simulink model "Template_v3_08_2020a"  (R2020a)
settings: Solver=FixedStepAuto  StartTime=0.0  StopTime=tsim  FixedStep=baseRate  MaxStep=0.0001  RelTol=1e-6  AbsTol=1e-6  EnableMultiTasking=on
values from neighbouring files (symbols this model uses):
  baseRate = 0.05    [Run_Initializer.m]
  drop_states_ARM = [ pi/2, pi/2, 0]    [Run_Initializer.m]
  drop_states_BLACK = [ xLength/2, yLength/2, 0]    [Run_Initializer.m]
  drop_states_BLUE = [ xLength/2-0.5; yLength/2; 0]    [Run_Initializer.m]
  drop_states_RED = [ xLength/2+0.5, yLength/2, pi]    [Run_Initializer.m]
  F_Black_X_nominal = 0.2196    [Run_Initializer.m]
  F_Black_Y_nominal = 0.2825    [Run_Initializer.m]
  F_Blue_X_nominal = 0.2196    [Run_Initializer.m]
  F_Blue_Y_nominal = 0.2825    [Run_Initializer.m]
  F_red_X_nominal = 0.2196    [Run_Initializer.m]
  F_red_Y_nominal = 0.2825    [Run_Initializer.m]
  F_thrusters_BLACK = [F_Black_X_nominal; F_Black_X_nominal;                             F_Black_Y_nominal; F_Black_Y_nominal; F_Black_X_nominal;                              F_Black_X_nominal; F_Black_Y_nominal; F_Black_Y_nominal]    [Run_Initializer.m]
  F_thrusters_BLUE = [F_Blue_X_nominal; F_Blue_X_nominal;                             F_Blue_Y_nominal; F_Blue_Y_nominal; F_Blue_X_nominal;                              F_Blue_X_nominal; F_Blue_Y_nominal; F_Blue_Y_nominal]    [Run_Initializer.m]
  F_thrusters_RED = [F_red_X_nominal; F_red_X_nominal;                             F_red_Y_nominal; F_red_Y_nominal; F_red_X_nominal;                              F_red_X_nominal; F_red_Y_nominal; F_red_Y_nominal]    [Run_Initializer.m]
  Gamma1_el = 0.12    [Run_Initializer.m]
  Gamma1_sh = 0.005    [Run_Initializer.m]
  Gamma1_wr = 0.025    [Run_Initializer.m]
  Gamma2_el = 5    [Run_Initializer.m]
  Gamma2_sh = 15    [Run_Initializer.m]
  Gamma2_wr = 5    [Run_Initializer.m]
  Gamma3_el = 10    [Run_Initializer.m]
  Gamma3_sh = 40    [Run_Initializer.m]
  Gamma3_wr = 40    [Run_Initializer.m]
  Gamma4_el = 0.039    [Run_Initializer.m]
  Gamma4_sh = 0.015    [Run_Initializer.m]
  Gamma4_wr = 0.029    [Run_Initializer.m]
  Gamma5_el = 800    [Run_Initializer.m]
  Gamma5_sh = 800    [Run_Initializer.m]
  Gamma5_wr = 800    [Run_Initializer.m]
  Gamma6_el = 0.000001    (= 1e-06)    [Run_Initializer.m]
  Gamma6_sh = 0.005    [Run_Initializer.m]
  Gamma6_wr = 0.02    [Run_Initializer.m]
  home_states_BLACK = [ xLength/2; yLength/2; 0]    [Run_Initializer.m]
  home_states_BLUE = [ xLength/2-0.9; yLength/2; 0]    [Run_Initializer.m]
  home_states_RED = [ xLength/2+0.9; yLength/2; pi]    [Run_Initializer.m]
  init_states_BLACK = [ xLength/2; yLength/2; 0]    [Run_Initializer.m]
  init_states_BLUE = [ xLength/2-0.9; yLength/2; 0]    [Run_Initializer.m]
  init_states_RED = [ xLength/2+0.9; yLength/2; pi]    [Run_Initializer.m]
  Kd_tb = 1.0    (= 1)    [Run_Initializer.m]
  Kd_tblue = 1    [Run_Initializer.m]
  Kd_tr = 1.0    (= 1)    [Run_Initializer.m]
  Kd_xb = 8    [Run_Initializer.m]
  Kd_xblue = 8    [Run_Initializer.m]
  Kd_xr = 8    [Run_Initializer.m]
  Kd_yb = 8    [Run_Initializer.m]
  Kd_yblue = 8    [Run_Initializer.m]
  Kd_yr = 8    [Run_Initializer.m]
  Kp_tb = 0.1    [Run_Initializer.m]
  Kp_tblue = 0.1    [Run_Initializer.m]
  Kp_tr = 0.1    [Run_Initializer.m]
  Kp_xb = 2    [Run_Initializer.m]
  Kp_xblue = 2    [Run_Initializer.m]
  Kp_xr = 2    [Run_Initializer.m]
  Kp_yb = 2    [Run_Initializer.m]
  Kp_yblue = 2    [Run_Initializer.m]
  Kp_yr = 2    [Run_Initializer.m]
  noise_variance_BLACK = 0    [Run_Initializer.m]
  noise_variance_BLUE = 0    [Run_Initializer.m]
  noise_variance_RED = 0    [Run_Initializer.m]
  Phase0_End = Phase0_Duration    (= 10)    [Run_Initializer.m]
  Phase1_End = Phase0_Duration + Phase1_Duration    (= 15)    [Run_Initializer.m]
  Phase2_End = Phase0_Duration + Phase1_Duration +                                   Phase2_Duration    (= 35)    [Run_Initializer.m]
  Phase3_End = Phase0_Duration + Phase1_Duration +                                   Phase2_Duration + Phase3_Duration    (= 155)    [Run_Initializer.m]
  Phase3_SubPhase1_End = Phase2_End + Phase3_SubPhase1_Duration    (= 155)    [Run_Initializer.m]
  Phase3_SubPhase2_End = Phase2_End + Phase3_SubPhase1_Duration +                                   Phase3_SubPhase2_Duration    (= 155)    [Run_Initializer.m]
  Phase3_SubPhase3_End = Phase2_End + Phase3_SubPhase1_Duration +                                   Phase3_SubPhase2_Duration +                                  Phase3_SubPhase3_Duration    (= 155)    [Run_Initializer.m]
  Phase3_SubPhase4_End = Phase2_End + Phase3_SubPhase1_Duration +                                   Phase3_SubPhase2_Duration +                                  Phase3_SubPhase3_Duration +                                  Phase3_SubPhase4_Duration    [Run_Initializer.m]
  Phase4_End = Phase0_Duration + Phase1_Duration +                                   Phase2_Duration + Phase3_Duration +                                   Phase4_Duration    (= 275)    [Run_Initializer.m]
  Phase5_End = Phase0_Duration + Phase1_Duration +                                   Phase2_Duration + Phase3_Duration +                                   Phase4_Duration + Phase5_Duration    (= 295)    [Run_Initializer.m]
  thruster_dist2CG_BLACK = [72.80;-65.20;61.75;-79.75;65.20;-65.20;74.25;-54.75]    [Run_Initializer.m]
  thruster_dist2CG_BLUE = [83.10;-54.90;71.50;-70.00;54.90;-75.50;64.50;-64.50]    [Run_Initializer.m]
  thruster_dist2CG_RED = [69.38;-56.62;50.01;-81.49;61.12;-68.38;78.99;-52.01]    [Run_Initializer.m]
  Tz_lim_elarm = .1    (= 0.1)    [Run_Initializer.m]
  Tz_lim_sharm = .1    (= 0.1)    [Run_Initializer.m]
  Tz_lim_wrarm = .1    (= 0.1)    [Run_Initializer.m]
  xLength = 3.51155    [Run_Initializer.m]
  yLength = 2.41935    [Run_Initializer.m]
undefined symbols (not defined in the file or in its folder): b0, b1, b_out, CHASER_ABSOLUTE_POSITION, DiscIntNeverNeededParam, MAX_BODY_ANGULAR_VELOCITY, MAX_VELOCITY, model_param, platformSelection, relevant_half_range, relevant_state_mean, serverRate, simMode, w0, w1, w_out
libraries: dspstat3 x18, raspberrypiBasiclib x9, dspsigops x9, embdlinuxlib x7, simulink x7, MainLibrary x4, mspfiltlib x3, dsparch4 x3, etargetslib x1, sensehatlib x1
(part 3 of 12)

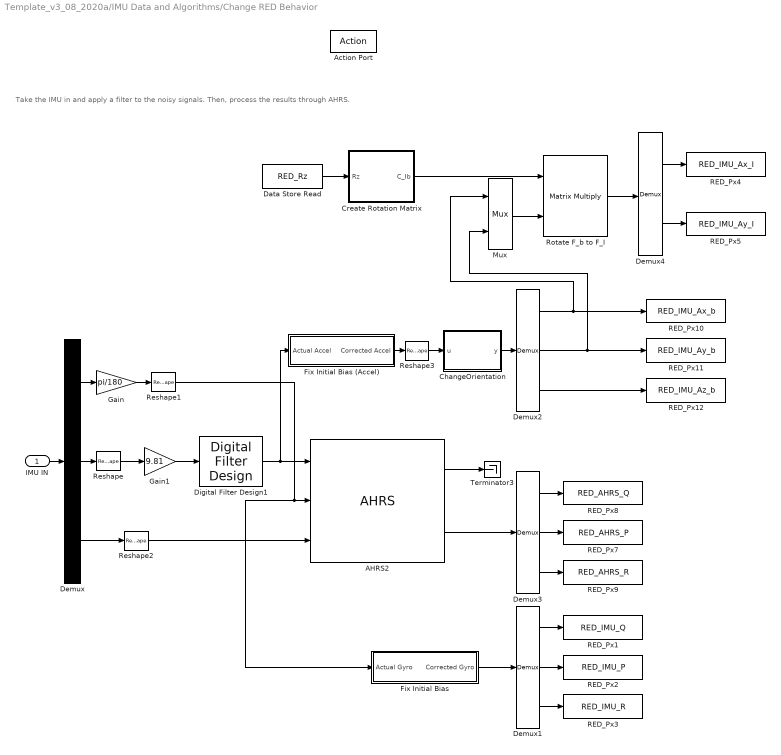
== system Template_v3_08_2020a/IMU Data and Algorithms/Change RED Behavior ==
  note: Take the IMU in and apply a filter to the noisy signals. Then, process the results through AHRS.
  IMU IN : Inport
  Action Port : ActionPort  ActionPortLabel=if(u1 == 1 & u2 ==0)
  AHRS2 : mspfiltlib/AHRS  DispRefFrame=NED  DecimationFactor=1  InitialProcessNoise=ahrsfilter.defaultProcessNoise  OrientationFormat=quaternion  SimulateUsing=Interpreted execution  AccelerometerNoise=0.0001924722  GyroscopeNoise=9.1385e-5  MagnetometerNoise=0.1  GyroscopeDriftNoise=3.0462e-13  LinearAccelerationNoise=0.0096236100000000012  MagneticDisturbanceNoise=0.5  LinearAccelerationDecayFactor=0.5  MagneticDisturbanceDecayFactor=0.5  ExpectedMagneticFieldStrength=33
      settings: SourceProductBaseCode=TF,NV
  ChangeOrientation : MATLAB Function  TreatAsAtomicUnit=on
  Create Rotation Matrix : MATLAB Function  TreatAsAtomicUnit=on
  Data Store Read : DataStoreRead  DataStoreName=RED_Rz
  Demux : Demux  Outputs=[3,3,3]
  Demux1 : Demux  Outputs=3
  Demux2 : Demux  Outputs=3
  Demux3 : Demux  Outputs=3
  Demux4 : Demux  Outputs=2
  Digital Filter Design1 : dsparch4/Digital Filter Design  mwdsp_browser_bugfix_var=off
  Fix Initial Bias : Subsystem
  Fix Initial Bias (Accel) : Subsystem
  Gain : Gain  Gain=pi/180
  Gain1 : Gain  Gain=9.81
  Mux : Mux  Inputs=2
  RED_Px1 : DataStoreWrite  DataStoreName=RED_IMU_Q
  RED_Px10 : DataStoreWrite  DataStoreName=RED_IMU_Ax_b
  RED_Px11 : DataStoreWrite  DataStoreName=RED_IMU_Ay_b
  RED_Px12 : DataStoreWrite  DataStoreName=RED_IMU_Az_b
  RED_Px2 : DataStoreWrite  DataStoreName=RED_IMU_P
  RED_Px3 : DataStoreWrite  DataStoreName=RED_IMU_R
  RED_Px4 : DataStoreWrite  DataStoreName=RED_IMU_Ax_I
  RED_Px5 : DataStoreWrite  DataStoreName=RED_IMU_Ay_I
  RED_Px7 : DataStoreWrite  DataStoreName=RED_AHRS_P
  RED_Px8 : DataStoreWrite  DataStoreName=RED_AHRS_Q
  RED_Px9 : DataStoreWrite  DataStoreName=RED_AHRS_R
  Reshape{,1..3} (4 alike) : Reshape  OutputDimensionality=Row vector (2-D)
  Rotate F_b to F_I : Product  Multiplication=Matrix(*)
  Terminator3 : Terminator
  wires:
  Reshape2/1 -> AHRS2/3
  Gain/1 -> Reshape1/1
  Demux2/3 -> RED_Px12/1
  Demux3/3 -> RED_Px9/1
  AHRS2/2 -> Demux3/1
  AHRS2/1 -> Terminator3/1
  Reshape/1 -> Gain1/1
  Demux/2 -> Reshape/1
  Demux/3 -> Reshape2/1
  Demux/1 -> Gain/1
  IMU IN/1 -> Demux/1
  Demux1/1 -> RED_Px1/1
  Demux1/2 -> RED_Px2/1
  Demux1/3 -> RED_Px3/1
  Fix Initial Bias/1(Corrected Gyro) -> Demux1/1
  ChangeOrientation/1(y) -> Demux2/1
  Demux3/2 -> RED_Px7/1
  Demux3/1 -> RED_Px8/1
  Digital Filter Design1/1 -> Fix Initial Bias (Accel)/1(Actual Accel), AHRS2/1
  Gain1/1 -> Digital Filter Design1/1
  Reshape3/1 -> ChangeOrientation/1(u)
  Fix Initial Bias (Accel)/1(Corrected Accel) -> Reshape3/1
  Reshape1/1 -> Fix Initial Bias/1(Actual Gyro), AHRS2/2
  Data Store Read/1 -> Create Rotation Matrix/1(Rz)
  Mux/1 -> Rotate F_b to F_I/2
  Rotate F_b to F_I/1 -> Demux4/1
  Create Rotation Matrix/1(C_Ib) -> Rotate F_b to F_I/1
  Demux2/2 -> Mux/2, RED_Px11/1
  Demux4/1 -> RED_Px4/1
  Demux4/2 -> RED_Px5/1
  Demux2/1 -> Mux/1, RED_Px10/1

== system Template_v3_08_2020a/IMU Data and Algorithms/Is this a simulation? ==
  Constant : Constant  Value=simMode  SampleTime=-1
  isSim : Outport  VectorParamsAs1DForOutWhenUnconnected=off
  wires:
  Constant/1 -> isSim/1

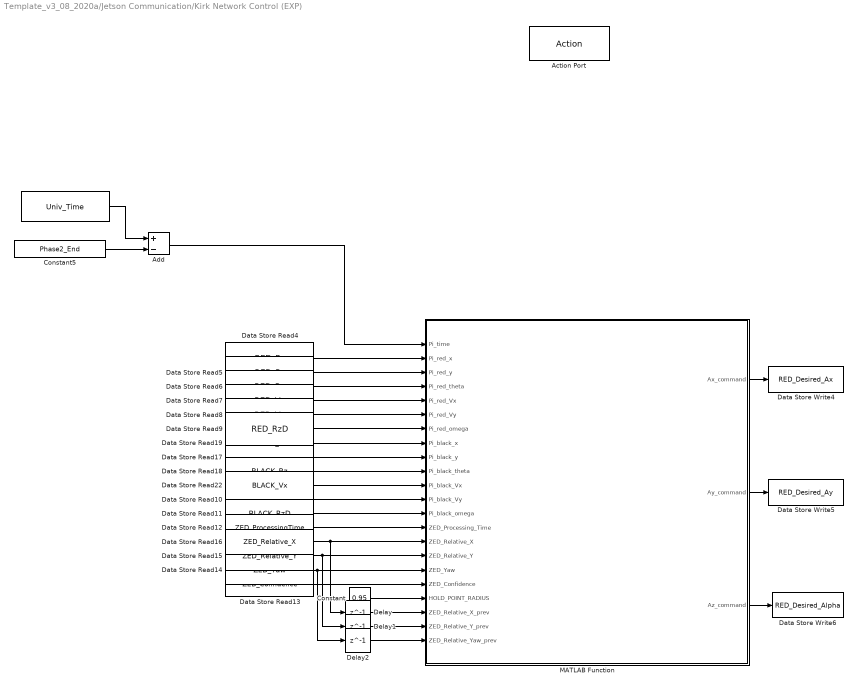
== system Template_v3_08_2020a/Jetson Communication/Kirk Network Control (EXP) ==
  Action Port : ActionPort  ActionPortLabel=if((u1 == 1 & u2 == 0) & (u3 > u4) & (u3 < u5) )
  " " : DataStoreRead  DataStoreName=Univ_Time
  Add : Sum  Inputs=+-
  Constant : Constant  Value=0.95
  Constant5 : Constant  Value=Phase2_End
  Data Store Read10 : DataStoreRead  DataStoreName=BLACK_Vy
  Data Store Read11 : DataStoreRead  DataStoreName=BLACK_RzD
  Data Store Read12 : DataStoreRead  DataStoreName=ZED_ProcessingTime
  Data Store Read13 : DataStoreRead  DataStoreName=ZED_Confidence
  Data Store Read14 : DataStoreRead  DataStoreName=ZED_Yaw
  Data Store Read15 : DataStoreRead  DataStoreName=ZED_Relative_Y
  Data Store Read16 : DataStoreRead  DataStoreName=ZED_Relative_X
  Data Store Read17 : DataStoreRead  DataStoreName=BLACK_Py
  Data Store Read18 : DataStoreRead  DataStoreName=BLACK_Rz
  Data Store Read19 : DataStoreRead  DataStoreName=BLACK_Px
  Data Store Read22 : DataStoreRead  DataStoreName=BLACK_Vx
  Data Store Read4 : DataStoreRead  DataStoreName=RED_Px
  Data Store Read5 : DataStoreRead  DataStoreName=RED_Py
  Data Store Read6 : DataStoreRead  DataStoreName=RED_Rz
  Data Store Read7 : DataStoreRead  DataStoreName=RED_Vx
  Data Store Read8 : DataStoreRead  DataStoreName=RED_Vy
  Data Store Read9 : DataStoreRead  DataStoreName=RED_RzD
  Data Store Write4 : DataStoreWrite  DataStoreName=RED_Desired_Ax
  Data Store Write5 : DataStoreWrite  DataStoreName=RED_Desired_Ay
  Data Store Write6 : DataStoreWrite  DataStoreName=RED_Desired_Alpha
  Delay : Delay  DelayLength=1
  Delay1 : Delay  DelayLength=1
  Delay2 : Delay  DelayLength=1
  MATLAB Function : MATLAB Function  TreatAsAtomicUnit=on
  wires:
  Data Store Read11/1 -> MATLAB Function/13(Pi_black_omega)
  Data Store Read7/1 -> MATLAB Function/5(Pi_red_Vx)
  " "/1 -> Add/1
  Data Store Read18/1 -> MATLAB Function/10(Pi_black_theta)
  Data Store Read17/1 -> MATLAB Function/9(Pi_black_y)
  Data Store Read8/1 -> MATLAB Function/6(Pi_red_Vy)
  MATLAB Function/2(Ay_command) -> Data Store Write5/1
  Data Store Read10/1 -> MATLAB Function/12(Pi_black_Vy)
  Data Store Read22/1 -> MATLAB Function/11(Pi_black_Vx)
  Data Store Read19/1 -> MATLAB Function/8(Pi_black_x)
  Data Store Read5/1 -> MATLAB Function/3(Pi_red_y)
  Add/1 -> MATLAB Function/1(Pi_time)
  Data Store Read9/1 -> MATLAB Function/7(Pi_red_omega)
  Constant5/1 -> Add/2
  Data Store Read15/1 -> MATLAB Function/16(ZED_Relative_Y), Delay1/1
  Data Store Read13/1 -> MATLAB Function/18(ZED_Confidence)
  MATLAB Function/3(Az_command) -> Data Store Write6/1
  Data Store Read12/1 -> MATLAB Function/14(ZED_Processing_Time)
  MATLAB Function/1(Ax_command) -> Data Store Write4/1
  Data Store Read6/1 -> MATLAB Function/4(Pi_red_theta)
  Data Store Read4/1 -> MATLAB Function/2(Pi_red_x)
  Data Store Read16/1 -> Delay/1, MATLAB Function/15(ZED_Relative_X)
  Data Store Read14/1 -> Delay2/1, MATLAB Function/17(ZED_Yaw)
  Constant/1 -> MATLAB Function/19(HOLD_POINT_RADIUS)
  Delay/1 -> MATLAB Function/20(ZED_Relative_X_prev)
  Delay1/1 -> MATLAB Function/21(ZED_Relative_Y_prev)
  Delay2/1 -> MATLAB Function/22(ZED_Relative_Yaw_prev)

== system Template_v3_08_2020a/Jetson Communication/Kirk Network Control (SIM) ==
  Action Port : ActionPort  ActionPortLabel=elseif((u2 == 1) & (u3 > u4) & (u3 < u5) )
  " " : DataStoreRead  DataStoreName=Univ_Time
  Add : Sum  Inputs=+-
  Constant : Constant  Value=0.95
  Constant5 : Constant  Value=Phase2_End
  Data Store Read : DataStoreRead  DataStoreName=RED_Px
  Data Store Read1 : DataStoreRead  DataStoreName=RED_Py
  Data Store Read10 : DataStoreRead  DataStoreName=BLACK_Vy
  Data Store Read11 : DataStoreRead  DataStoreName=BLACK_RzD
  Data Store Read17 : DataStoreRead  DataStoreName=BLACK_Py
  Data Store Read18 : DataStoreRead  DataStoreName=BLACK_Rz
  Data Store Read2 : DataStoreRead  DataStoreName=RED_Rz
  Data Store Read22 : DataStoreRead  DataStoreName=BLACK_Vx
  Data Store Read6 : DataStoreRead  DataStoreName=RED_Vx
  Data Store Read7 : DataStoreRead  DataStoreName=RED_Vy
  Data Store Read8 : DataStoreRead  DataStoreName=RED_RzD
  Data Store Read9 : DataStoreRead  DataStoreName=BLACK_Px
  Data Store Write3 : DataStoreWrite  DataStoreName=RED_Desired_Ax
  Data Store Write4 : DataStoreWrite  DataStoreName=RED_Desired_Ay
  Data Store Write5 : DataStoreWrite  DataStoreName=RED_Desired_Alpha
  Delay : Delay  DelayLength=10
  Delay1 : Delay  DelayLength=10
  Delay2 : Delay  DelayLength=10
  MATLAB Function : MATLAB Function  TreatAsAtomicUnit=on
  Zero-Order Hold : ZeroOrderHold  SampleTime=0.5
  Zero-Order Hold1 : ZeroOrderHold  SampleTime=0.5
  Zero-Order Hold2 : ZeroOrderHold  SampleTime=0.5
  wires:
  Data Store Read1/1 -> MATLAB Function/3(Pi_red_y)
  Data Store Read/1 -> MATLAB Function/2(Pi_red_x)
  Data Store Read2/1 -> MATLAB Function/4(Pi_red_theta)
  Data Store Read9/1 -> Zero-Order Hold/1
  Data Store Read17/1 -> Zero-Order Hold1/1
  Data Store Read18/1 -> Zero-Order Hold2/1
  MATLAB Function/1(Ax_command) -> Data Store Write3/1
  MATLAB Function/2(Ay_command) -> Data Store Write4/1
  MATLAB Function/3(Az_command) -> Data Store Write5/1
  Data Store Read6/1 -> MATLAB Function/5(Pi_red_Vx)
  Data Store Read7/1 -> MATLAB Function/6(Pi_red_Vy)
  Data Store Read8/1 -> MATLAB Function/7(Pi_red_omega)
  Data Store Read22/1 -> MATLAB Function/11(Pi_black_Vx)
  Data Store Read10/1 -> MATLAB Function/12(Pi_black_Vy)
  Data Store Read11/1 -> MATLAB Function/13(Pi_black_omega)
  " "/1 -> Add/1
  Add/1 -> MATLAB Function/1(Pi_time)
  Constant5/1 -> Add/2
  Zero-Order Hold/1 -> Delay/1
  Zero-Order Hold1/1 -> Delay1/1
  Zero-Order Hold2/1 -> Delay2/1
  Constant/1 -> MATLAB Function/14(HOLD_POINT_RADIUS)
  Delay/1 -> MATLAB Function/8(Pi_black_x)
  Delay1/1 -> MATLAB Function/9(Pi_black_y)
  Delay2/1 -> MATLAB Function/10(Pi_black_theta)

== system Template_v3_08_2020a/Jetson Communication/isSim ==
  Constant : Constant  Value=simMode  SampleTime=-1
  isSim : Outport  VectorParamsAs1DForOutWhenUnconnected=off
  wires:
  Constant/1 -> isSim/1

== system Template_v3_08_2020a/Manipulator Encoder Data/Change Behavior ==
  Action Port : ActionPort  ActionPortLabel=if(u1 == 0)
  Data Store Write : DataStoreWrite  DataStoreName=RED_Rz_Shoulder
  Data Store Write1 : DataStoreWrite  DataStoreName=RED_Rz_Elbow
  Data Store Write2 : DataStoreWrite  DataStoreName=RED_Rz_Wrist
  Data Store Write3 : DataStoreWrite  DataStoreName=RED_RzD_Shoulder
  Data Store Write4 : DataStoreWrite  DataStoreName=RED_RzD_Elbow
  Data Store Write5 : DataStoreWrite  DataStoreName=RED_RzD_Wrist
  Read Joint Positions using Dynamixel Encoders : MainLibrary/Dynamixel Functions/Read Joint Positions using  Dynamixel Encoders  SampleTime=baseRate
      settings: SourceProductName=SPOT Custom Library
  wires:
  Read Joint Positions using Dynamixel Encoders/1 -> Data Store Write/1
  Read Joint Positions using Dynamixel Encoders/2 -> Data Store Write1/1
  Read Joint Positions using Dynamixel Encoders/3 -> Data Store Write2/1
  Read Joint Positions using Dynamixel Encoders/4 -> Data Store Write3/1
  Read Joint Positions using Dynamixel Encoders/5 -> Data Store Write4/1
  Read Joint Positions using Dynamixel Encoders/6 -> Data Store Write5/1

== system Template_v3_08_2020a/Manipulator Encoder Data/Is this a simulation? ==
  Constant : Constant  Value=simMode  SampleTime=-1
  isSim : Outport  VectorParamsAs1DForOutWhenUnconnected=off
  wires:
  Constant/1 -> isSim/1

== system Template_v3_08_2020a/Phase #0: Wait for Synchronization/Change BLACK Behavior ==
  note: Before getting good data, the platforms must NOT be floating. So, float is set to be "off".
  note: For the initialization phase, we do not want any thrust. Thus, all commanded forces are zero.
  Action Port : ActionPort  ActionPortLabel=if(u1 == 2 | u2 == 1)
  BLACK_Fx : DataStoreWrite  DataStoreName=BLACK_Fx
  BLACK_Fy : DataStoreWrite  DataStoreName=BLACK_Fy
  BLACK_Tz : DataStoreWrite  DataStoreName=BLACK_Tz
  Constant1 : Constant
  Constant3 : Constant  Value=0
  Constant4 : Constant  Value=0
  Constant5 : Constant  Value=0
  Data Store Write : DataStoreWrite  DataStoreName=Magnet_State
  Data Store Write4 : DataStoreWrite  DataStoreName=Float_State
  Puck State : Constant  Value=0
  wires:
  Constant3/1 -> BLACK_Fx/1
  Constant5/1 -> BLACK_Tz/1
  Constant4/1 -> BLACK_Fy/1
  Puck State/1 -> Data Store Write4/1
  Constant1/1 -> Data Store Write/1

== system Template_v3_08_2020a/Phase #0: Wait for Synchronization/Change BLUE Behavior ==
  note: Before getting good data, the platforms must NOT be floating. So, float is set to be "off".
  note: For the initialization phase, we do not want any thrust. Thus, all commanded forces are zero.
  Action Port : ActionPort  ActionPortLabel=if(u1 == 3 | u2 == 1)
  BLUE_Fx : DataStoreWrite  DataStoreName=BLUE_Fx
  BLUE_Fy : DataStoreWrite  DataStoreName=BLUE_Fy
  BLUE_Tz : DataStoreWrite  DataStoreName=BLUE_Tz
  Constant3 : Constant  Value=0
  Constant4 : Constant  Value=0
  Constant5 : Constant  Value=0
  Data Store Write4 : DataStoreWrite  DataStoreName=Float_State
  Puck State : Constant  Value=0
  wires:
  Constant3/1 -> BLUE_Fx/1
  Constant5/1 -> BLUE_Tz/1
  Constant4/1 -> BLUE_Fy/1
  Puck State/1 -> Data Store Write4/1

== system Template_v3_08_2020a/Phase #0: Wait for Synchronization/Change RED Behavior ==
  note: For the initialization phase, we do not want any thrust or movement from the robotic arm. Thus, all commanded forces are zero.
  note: Before getting good data, the platforms must NOT be floating. So, float is set to be "off".
  Action Port : ActionPort  ActionPortLabel=if(u1 == 1 | u2 == 1)
  Constant{,1..3,6..7} (6 alike) : Constant  Value=0
  Constant4 : Constant  Value=pi/2
  Constant5 : Constant  Value=pi/2
  Data Store Write : DataStoreWrite  DataStoreName=RED_Shoulder_Command
  Data Store Write1 : DataStoreWrite  DataStoreName=RED_Elbow_Command
  Data Store Write2 : DataStoreWrite  DataStoreName=RED_Wrist_Command
  Data Store Write3 : DataStoreWrite  DataStoreName=RED_ARM_Control_Mode
  Data Store Write4 : DataStoreWrite  DataStoreName=Float_State
  Puck State : Constant  Value=0
  RED_Fx : DataStoreWrite  DataStoreName=RED_Fx
  RED_Fy : DataStoreWrite  DataStoreName=RED_Fy
  RED_Tz : DataStoreWrite  DataStoreName=RED_Tz
  RED_Tz_RW : DataStoreWrite  DataStoreName=RED_Tz_RW
  wires:
  Constant1/1 -> RED_Fy/1
  Constant2/1 -> RED_Tz/1
  Constant/1 -> RED_Fx/1
  Constant4/1 -> Data Store Write/1
  Constant5/1 -> Data Store Write1/1
  Constant6/1 -> Data Store Write2/1
  Constant3/1 -> RED_Tz_RW/1
  Puck State/1 -> Data Store Write4/1
  Constant7/1 -> Data Store Write3/1

== system Template_v3_08_2020a/Phase #0: Wait for Synchronization/Is this a simulation? ==
  Constant : Constant  Value=simMode  SampleTime=-1
  isSim : Outport  VectorParamsAs1DForOutWhenUnconnected=off
  wires:
  Constant/1 -> isSim/1

== system Template_v3_08_2020a/Phase #1: Start Floating /Change BLACK Behavior ==
  note: For the float phase, we do not want any thrust. Thus, all commanded forces are zero.
  note: Now that good data is available, the platform can start to float.
  Action Port : ActionPort  ActionPortLabel=if(u1 == 2 | u2 == 1)
  BLACK_Fx : DataStoreWrite  DataStoreName=BLACK_Fx
  BLACK_Fy : DataStoreWrite  DataStoreName=BLACK_Fy
  BLACK_Tz : DataStoreWrite  DataStoreName=BLACK_Tz
  Constant1 : Constant
  Constant3 : Constant  Value=0
  Constant4 : Constant  Value=0
  Constant5 : Constant  Value=0
  Data Store Write : DataStoreWrite  DataStoreName=Magnet_State
  Data Store Write4 : DataStoreWrite  DataStoreName=Float_State
  Puck State : Constant
  wires:
  Constant3/1 -> BLACK_Fx/1
  Constant5/1 -> BLACK_Tz/1
  Constant4/1 -> BLACK_Fy/1
  Puck State/1 -> Data Store Write4/1
  Constant1/1 -> Data Store Write/1

== system Template_v3_08_2020a/Phase #1: Start Floating /Change BLUE Behavior ==
  note: Before getting good data, the platforms must NOT be floating. So, float is set to be "off".
  note: For the initialization phase, we do not want any thrust. Thus, all commanded forces are zero.
  Action Port : ActionPort  ActionPortLabel=if(u1 == 3 | u2 == 1)
  BLUE_Fx : DataStoreWrite  DataStoreName=BLUE_Fx
  BLUE_Fy : DataStoreWrite  DataStoreName=BLUE_Fy
  BLUE_Tz : DataStoreWrite  DataStoreName=BLUE_Tz
  Constant3 : Constant  Value=0
  Constant4 : Constant  Value=0
  Constant5 : Constant  Value=0
  Data Store Write4 : DataStoreWrite  DataStoreName=Float_State
  Puck State : Constant
  wires:
  Constant3/1 -> BLUE_Fx/1
  Constant5/1 -> BLUE_Tz/1
  Constant4/1 -> BLUE_Fy/1
  Puck State/1 -> Data Store Write4/1

== system Template_v3_08_2020a/Phase #1: Start Floating /Change RED Behavior ==
  note: Now that good data is available, the platforms can start to float.
  note: For the float phase, we do not want any thrust or movement from the robotic arm. Thus, all commanded forces are zero.
  note: Calculate desired angular velocity based on commanded torque.
  Action Port : ActionPort  ActionPortLabel=if(u1 == 1 | u2 == 1)
  Constant{,1..3,6} (5 alike) : Constant  Value=0
  Constant4 : Constant  Value=pi/2
  Constant5 : Constant  Value=pi/2
  Constant7 : Constant
  Data Store Write : DataStoreWrite  DataStoreName=RED_Shoulder_Command
  Data Store Write1 : DataStoreWrite  DataStoreName=RED_Elbow_Command
  Data Store Write2 : DataStoreWrite  DataStoreName=RED_Wrist_Command
  Data Store Write3 : DataStoreWrite  DataStoreName=RED_ARM_Control_Mode
  Data Store Write4 : DataStoreWrite  DataStoreName=Float_State
  Puck State : Constant
  RED_Fx : DataStoreWrite  DataStoreName=RED_Fx
  RED_Fy : DataStoreWrite  DataStoreName=RED_Fy
  RED_Tz : DataStoreWrite  DataStoreName=RED_Tz
  RED_Tz_RW : DataStoreWrite  DataStoreName=RED_Tz_RW
  wires:
  Constant/1 -> RED_Fx/1
  Constant3/1 -> RED_Tz_RW/1
  Constant2/1 -> RED_Tz/1
  Constant1/1 -> RED_Fy/1
  Puck State/1 -> Data Store Write4/1
  Constant7/1 -> Data Store Write3/1
  Constant6/1 -> Data Store Write2/1
  Constant4/1 -> Data Store Write/1
  Constant5/1 -> Data Store Write1/1

== system Template_v3_08_2020a/Phase #1: Start Floating /Is this a simulation? ==
  Constant : Constant  Value=simMode  SampleTime=-1
  isSim : Outport  VectorParamsAs1DForOutWhenUnconnected=off
  wires:
  Constant/1 -> isSim/1

== system Template_v3_08_2020a/Phase #2: Move to Initial Position/Change BLACK Behavior ==
  note: Additional Blocks
  note: PD Control Law - BLACK
  note: Additional blocks are stored here.
  note: A simple PD control law is used here to command the platform to it's initial position, as defined in the initializer.
  Action Port : ActionPort  ActionPortLabel=if(u1 == 2 | u2 == 1)
  BLACK_Fx : DataStoreWrite  DataStoreName=BLACK_Fx
  BLACK_Fy : DataStoreWrite  DataStoreName=BLACK_Fy
  BLACK_Px : DataStoreRead  DataStoreName=BLACK_Px
  "BLACK_Py " : DataStoreRead  DataStoreName=BLACK_Py
  BLACK_Rz : DataStoreRead  DataStoreName=BLACK_Rz
  BLACK_Tz : DataStoreWrite  DataStoreName=BLACK_Tz
  Constant1 : Constant
  Custom Discrete PD (Attitude) : Subsystem
  Custom Discrete PD (X-Position) : Subsystem
  Custom Discrete PD (Y-Position) : Subsystem
  Data Store Write : DataStoreWrite  DataStoreName=Magnet_State
  Data Store Write3 : DataStoreWrite  DataStoreName=Float_State
  Desired Attitude (BLACK) : Constant  Value=init_states_BLACK(3)  SampleTime=-1
  Desired Px (BLACK) : Constant  Value=init_states_BLACK(1)  SampleTime=-1
  Desired Py (BLACK) : Constant  Value=init_states_BLACK(2)  SampleTime=-1
  Hough Control : Subsystem
  Puck State : Constant
  Subtract : Sum  Inputs=+-
  Subtract1 : Sum  Inputs=+-
  wires:
  Custom Discrete PD (Y-Position)/1(Fy) -> BLACK_Fy/1
  Hough Control/1(Err) -> Custom Discrete PD (Attitude)/1(ez)
  BLACK_Px/1 -> Subtract/2
  Subtract1/1 -> Custom Discrete PD (Y-Position)/1(ey)
  Custom Discrete PD (Attitude)/1(Tz) -> BLACK_Tz/1
  "BLACK_Py "/1 -> Subtract1/2
  Subtract/1 -> Custom Discrete PD (X-Position)/1(ex)
  Custom Discrete PD (X-Position)/1(Fx) -> BLACK_Fx/1
  Desired Px (BLACK)/1 -> Subtract/1
  Desired Py (BLACK)/1 -> Subtract1/1
  Desired Attitude (BLACK)/1 -> Hough Control/1(Ref)
  BLACK_Rz/1 -> Hough Control/2(Act)
  Puck State/1 -> Data Store Write3/1
  Constant1/1 -> Data Store Write/1

== system Template_v3_08_2020a/Phase #2: Move to Initial Position/Change BLUE Behavior ==
  note: PD Control Law - BLUE
  note: Additional blocks are stored here.
  note: A simple PD control law is used here to command the platform to it's initial position, as defined in the initializer.
  note: Additional Blocks
  Action Port : ActionPort  ActionPortLabel=if(u1 == 3 | u2 == 1)
  BLUE_Fx : DataStoreWrite  DataStoreName=BLUE_Fx
  BLUE_Fy : DataStoreWrite  DataStoreName=BLUE_Fy
  BLUE_Px : DataStoreRead  DataStoreName=BLUE_Px
  "BLUE_Py " : DataStoreRead  DataStoreName=BLUE_Py
  BLUE_Rz : DataStoreRead  DataStoreName=BLUE_Rz
  BLUE_Tz : DataStoreWrite  DataStoreName=BLUE_Tz
  Custom Discrete PD (Attitude) : Subsystem
  Custom Discrete PD (X-Position) : Subsystem
  Custom Discrete PD (Y-Position) : Subsystem
  Data Store Write3 : DataStoreWrite  DataStoreName=Float_State
  Desired Attitude (BLUE) : Constant  Value=init_states_BLUE(3)  SampleTime=-1
  Desired Px (BLUE) : Constant  Value=init_states_BLUE(1)  SampleTime=-1
  Desired Py (BLUE) : Constant  Value=init_states_BLUE(2)  SampleTime=-1
  Hough Control : Subsystem
  Puck State : Constant
  Subtract : Sum  Inputs=+-
  Subtract1 : Sum  Inputs=+-
  wires:
  Desired Attitude (BLUE)/1 -> Hough Control/1(Ref)
  BLUE_Rz/1 -> Hough Control/2(Act)
  Puck State/1 -> Data Store Write3/1
  Subtract/1 -> Custom Discrete PD (X-Position)/1(ex)
  Hough Control/1(Err) -> Custom Discrete PD (Attitude)/1(ez)
  Custom Discrete PD (X-Position)/1(Fx) -> BLUE_Fx/1
  Desired Py (BLUE)/1 -> Subtract1/1
  BLUE_Px/1 -> Subtract/2
  Subtract1/1 -> Custom Discrete PD (Y-Position)/1(ey)
  Desired Px (BLUE)/1 -> Subtract/1
  "BLUE_Py "/1 -> Subtract1/2
  Custom Discrete PD (Y-Position)/1(Fy) -> BLUE_Fy/1
  Custom Discrete PD (Attitude)/1(Tz) -> BLUE_Tz/1

== system Template_v3_08_2020a/Phase #2: Move to Initial Position/Change RED Behavior ==
  note: PD Control Law - RED
  note: Additional Blocks
  note: Additional blocks are stored above. Note that to control attitude using the RW, simply replace RED_Tz with RED_Tz_RW.
  note: A simple PD control law is used here to command the platform to it's initial position, as defined in the initializer.
  note: ARM Control Law - RED
  Action Port : ActionPort  ActionPortLabel=if(u1 == 1 | u2 == 1)
  Constant : Constant  Value=init_states_RED(3)
  Constant1 : Constant  Value=init_states_RED(1)
  Constant2 : Constant  Value=0
  Constant3 : Constant  Value=init_states_RED(2)
  Constant4 : Constant  Value=platformSelection
  Custom Discrete PD (Attitude) : Subsystem
  Custom Discrete PD (X-Position) : Subsystem
  Custom Discrete PD (Y-Position) : Subsystem
  Data Store Write3 : DataStoreWrite  DataStoreName=Float_State
  Hough Control : Subsystem
  If : If  IfExpression=u1 == 4 | u1 == 5 | u1 == 10 | u1 == 11
  Puck State : Constant
  RED : Subsystem  TreatAsAtomicUnit=on
  RED+ARM : Subsystem  TreatAsAtomicUnit=on
  RED_Fx : DataStoreWrite  DataStoreName=RED_Fx
  RED_Fy : DataStoreWrite  DataStoreName=RED_Fy
  RED_Px : DataStoreRead  DataStoreName=RED_Px
  "RED_Py " : DataStoreRead  DataStoreName=RED_Py
  RED_Rz : DataStoreRead  DataStoreName=RED_Rz
  RED_Tz : DataStoreWrite  DataStoreName=RED_Tz
  RED_Tz_RW1 : DataStoreWrite  DataStoreName=RED_Tz_RW
  Subtract : Sum  Inputs=+-
  Subtract1 : Sum  Inputs=+-
  wires:
  Constant2/1 -> RED_Tz_RW1/1
  Custom Discrete PD (Attitude)/1(Tz) -> RED_Tz/1
  RED_Rz/1 -> Hough Control/2(Act)
  Custom Discrete PD (X-Position)/1(Fx) -> RED_Fx/1
  Subtract/1 -> Custom Discrete PD (X-Position)/1(ex)
  Hough Control/1(Err) -> Custom Discrete PD (Attitude)/1(ez)
  Custom Discrete PD (Y-Position)/1(Fy) -> RED_Fy/1
  RED_Px/1 -> Subtract/2
  "RED_Py "/1 -> Subtract1/2
  Subtract1/1 -> Custom Discrete PD (Y-Position)/1(ey)
  Constant1/1 -> Subtract/1
  Constant3/1 -> Subtract1/1
  Constant/1 -> Hough Control/1(Ref)
  Puck State/1 -> Data Store Write3/1
  If/1 -> RED+ARM/Action
  If/2 -> RED/Action
  Constant4/1 -> If/1

== system Template_v3_08_2020a/Phase #2: Move to Initial Position/Is this a simulation? ==
  Constant : Constant  Value=simMode  SampleTime=-1
  isSim : Outport  VectorParamsAs1DForOutWhenUnconnected=off
  wires:
  Constant/1 -> isSim/1

== system Template_v3_08_2020a/Phase #3: Experiment/Change BLACK Behavior ==
  note: For experiments, it is usually desirable to have various sub-phases. The sub-phases are defined in the initializer; note that in the template only three sub-phases are present, but more can be added.
  Action Port : ActionPort  ActionPortLabel=if(u1 == 2 | u2 == 1)
  Constant1 : Constant  Value=Phase3_SubPhase2_End  SampleTime=-1
  Constant2 : Constant  Value=Phase3_SubPhase3_End  SampleTime=-1
  Constant3 : Constant  Value=Phase3_SubPhase4_End  SampleTime=-1
  Constant4 : Constant  Value=Phase3_SubPhase1_End  SampleTime=-1
  Experiment Sub-Phases : If  NumInputs=5  IfExpression=u1 < u2  ElseIfExpressions=u1 < u3, u1 < u4, u1 < u5  ShowElse=off
  Sub-Phase #1 : Subsystem  TreatAsAtomicUnit=on
  "Sub-Phase #2 " : Subsystem  TreatAsAtomicUnit=on
  "Sub-Phase #3 " : Subsystem  TreatAsAtomicUnit=on
  Sub-Phase #4 : Subsystem  TreatAsAtomicUnit=on
  Subsystem : Subsystem
  wires:
  Experiment Sub-Phases/2 -> "Sub-Phase #2 "/Action
  Experiment Sub-Phases/1 -> Sub-Phase #1/Action
  Experiment Sub-Phases/3 -> "Sub-Phase #3 "/Action
  Constant1/1 -> Experiment Sub-Phases/3
  Constant2/1 -> Experiment Sub-Phases/4
  Constant4/1 -> Experiment Sub-Phases/2
  Subsystem/1(Time) -> Experiment Sub-Phases/1
  Constant3/1 -> Experiment Sub-Phases/5
  Experiment Sub-Phases/4 -> Sub-Phase #4/Action

== system Template_v3_08_2020a/Phase #3: Experiment/Change BLUE Behavior ==
  Action Port : ActionPort  ActionPortLabel=if(u1 == 3 | u2 == 1)
  Constant1 : Constant  Value=Phase3_SubPhase2_End  SampleTime=-1
  Constant2 : Constant  Value=Phase3_SubPhase3_End  SampleTime=-1
  Constant3 : Constant  Value=Phase3_SubPhase4_End  SampleTime=-1
  Constant4 : Constant  Value=Phase3_SubPhase1_End  SampleTime=-1
  Experiment Sub-Phases : If  NumInputs=5  IfExpression=u1 < u2  ElseIfExpressions=u1 < u3, u1 < u4, u1 < u5  ShowElse=off
  Sub-Phase #1 : Subsystem  TreatAsAtomicUnit=on
  "Sub-Phase #2 " : Subsystem  TreatAsAtomicUnit=on
  "Sub-Phase #3 " : Subsystem  TreatAsAtomicUnit=on
  Sub-Phase #4 : Subsystem  TreatAsAtomicUnit=on
  Subsystem : Subsystem
  wires:
  Constant3/1 -> Experiment Sub-Phases/5
  Experiment Sub-Phases/4 -> Sub-Phase #4/Action
  Subsystem/1(Time) -> Experiment Sub-Phases/1
  Experiment Sub-Phases/1 -> Sub-Phase #1/Action
  Constant2/1 -> Experiment Sub-Phases/4
  Constant4/1 -> Experiment Sub-Phases/2
  Constant1/1 -> Experiment Sub-Phases/3
  Experiment Sub-Phases/3 -> "Sub-Phase #3 "/Action
  Experiment Sub-Phases/2 -> "Sub-Phase #2 "/Action

== system Template_v3_08_2020a/Phase #3: Experiment/Change RED Behavior ==
  note: For experiments, it is usually desirable to have various sub-phases. The sub-phases are defined in the initializer; note that in the template only three sub-phases are present, but more can be added.
  Action Port : ActionPort  ActionPortLabel=if(u1 == 1 | u2 == 1)
  Constant1 : Constant  Value=Phase3_SubPhase2_End  SampleTime=-1
  Constant2 : Constant  Value=Phase3_SubPhase3_End  SampleTime=-1
  Constant3 : Constant  Value=Phase3_SubPhase4_End  SampleTime=-1
  Constant4 : Constant  Value=Phase3_SubPhase1_End  SampleTime=-1
  Experiment Sub-Phases : If  NumInputs=5  IfExpression=u1 < u2  ElseIfExpressions=u1 < u3, u1 < u4, u1 < u5  ShowElse=off
  Sub-Phase #1 : Subsystem  TreatAsAtomicUnit=on
  "Sub-Phase #2 " : Subsystem  TreatAsAtomicUnit=on
  "Sub-Phase #3 " : Subsystem  TreatAsAtomicUnit=on
  Sub-Phase #4 : Subsystem  TreatAsAtomicUnit=on
  Subsystem : Subsystem
  wires:
  Experiment Sub-Phases/1 -> Sub-Phase #1/Action
  Experiment Sub-Phases/2 -> "Sub-Phase #2 "/Action
  Subsystem/1(Time) -> Experiment Sub-Phases/1
  Experiment Sub-Phases/3 -> "Sub-Phase #3 "/Action
  Constant4/1 -> Experiment Sub-Phases/2
  Constant1/1 -> Experiment Sub-Phases/3
  Constant2/1 -> Experiment Sub-Phases/4
  Constant3/1 -> Experiment Sub-Phases/5
  Experiment Sub-Phases/4 -> Sub-Phase #4/Action

== system Template_v3_08_2020a/Phase #3: Experiment/Is this a simulation? ==
  Constant : Constant  Value=simMode  SampleTime=-1
  isSim : Outport  VectorParamsAs1DForOutWhenUnconnected=off
  wires:
  Constant/1 -> isSim/1

== system Template_v3_08_2020a/Phase #4: Return Home/Change BLACK Behavior ==
  note: Additional Blocks
  note: PD Control Law - BLACK
  note: Additional blocks are stored here.
  note: A simple PD control law is used here to command the platform to it's initial position, as defined in the initializer.
  Action Port : ActionPort  ActionPortLabel=if(u1 == 2 | u2 == 1)
  BLACK_Fx : DataStoreWrite  DataStoreName=BLACK_Fx
  BLACK_Fy : DataStoreWrite  DataStoreName=BLACK_Fy
  BLACK_Px : DataStoreRead  DataStoreName=BLACK_Px
  "BLACK_Py " : DataStoreRead  DataStoreName=BLACK_Py
  BLACK_Rz : DataStoreRead  DataStoreName=BLACK_Rz
  BLACK_Tz : DataStoreWrite  DataStoreName=BLACK_Tz
  Constant1 : Constant
  Custom Discrete PD (Attitude) : Subsystem
  Custom Discrete PD (X-Position) : Subsystem
  Custom Discrete PD (Y-Position) : Subsystem
  Data Store Write : DataStoreWrite  DataStoreName=Magnet_State
  Data Store Write3 : DataStoreWrite  DataStoreName=Float_State
  Desired Attitude (BLACK) : Constant  Value=home_states_BLACK(3)  SampleTime=-1
  Desired Px (BLACK) : Constant  Value=home_states_BLACK(1)  SampleTime=-1
  Desired Py (BLACK) : Constant  Value=home_states_BLACK(2)  SampleTime=-1
  Hough Control : Subsystem
  Puck State : Constant
  Subtract : Sum  Inputs=+-
  Subtract1 : Sum  Inputs=+-
  wires:
  Custom Discrete PD (Y-Position)/1(Fy) -> BLACK_Fy/1
  Desired Py (BLACK)/1 -> Subtract1/1
  Hough Control/1(Err) -> Custom Discrete PD (Attitude)/1(ez)
  BLACK_Px/1 -> Subtract/2
  Subtract1/1 -> Custom Discrete PD (Y-Position)/1(ey)
  Custom Discrete PD (Attitude)/1(Tz) -> BLACK_Tz/1
  Desired Attitude (BLACK)/1 -> Hough Control/1(Ref)
  "BLACK_Py "/1 -> Subtract1/2
  Subtract/1 -> Custom Discrete PD (X-Position)/1(ex)
  BLACK_Rz/1 -> Hough Control/2(Act)
  Desired Px (BLACK)/1 -> Subtract/1
  Custom Discrete PD (X-Position)/1(Fx) -> BLACK_Fx/1
  Puck State/1 -> Data Store Write3/1
  Constant1/1 -> Data Store Write/1

== system Template_v3_08_2020a/Phase #4: Return Home/Change BLUE Behavior ==
  note: PD Control Law - BLUE
  note: Additional blocks are stored here.
  note: A simple PD control law is used here to command the platform to it's initial position, as defined in the initializer.
  note: Additional Blocks
  Action Port : ActionPort  ActionPortLabel=if(u1 == 3 | u2 == 1)
  BLUE_Fx : DataStoreWrite  DataStoreName=BLUE_Fx
  BLUE_Fy : DataStoreWrite  DataStoreName=BLUE_Fy
  BLUE_Px : DataStoreRead  DataStoreName=BLUE_Px
  "BLUE_Py " : DataStoreRead  DataStoreName=BLUE_Py
  BLUE_Rz : DataStoreRead  DataStoreName=BLUE_Rz
  BLUE_Tz : DataStoreWrite  DataStoreName=BLUE_Tz
  Custom Discrete PD (Attitude) : Subsystem
  Custom Discrete PD (X-Position) : Subsystem
  Custom Discrete PD (Y-Position) : Subsystem
  Data Store Write3 : DataStoreWrite  DataStoreName=Float_State
  Desired Attitude (BLUE) : Constant  Value=home_states_BLUE(3)  SampleTime=-1
  Desired Px (BLUE) : Constant  Value=home_states_BLUE(1)  SampleTime=-1
  Desired Py (BLUE) : Constant  Value=home_states_BLUE(2)  SampleTime=-1
  Hough Control : Subsystem
  Puck State : Constant
  Subtract : Sum  Inputs=+-
  Subtract1 : Sum  Inputs=+-
  wires:
  Puck State/1 -> Data Store Write3/1
  Subtract/1 -> Custom Discrete PD (X-Position)/1(ex)
  Desired Py (BLUE)/1 -> Subtract1/1
  Custom Discrete PD (X-Position)/1(Fx) -> BLUE_Fx/1
  Desired Px (BLUE)/1 -> Subtract/1
  Subtract1/1 -> Custom Discrete PD (Y-Position)/1(ey)
  Hough Control/1(Err) -> Custom Discrete PD (Attitude)/1(ez)
  Desired Attitude (BLUE)/1 -> Hough Control/1(Ref)
  Custom Discrete PD (Attitude)/1(Tz) -> BLUE_Tz/1
  "BLUE_Py "/1 -> Subtract1/2
  Custom Discrete PD (Y-Position)/1(Fy) -> BLUE_Fy/1
  BLUE_Px/1 -> Subtract/2
  BLUE_Rz/1 -> Hough Control/2(Act)

== system Template_v3_08_2020a/Phase #4: Return Home/Change RED Behavior ==
  note: PD Control Law - RED
  note: Additional Blocks
  note: Additional blocks are stored above. Note that to control attitude using the RW, simply replace RED_Tz with RED_Tz_RW.
  note: A simple PD control law is used here to command the platform to it's initial position, as defined in the initializer.
  note: ARM Control Law - RED
  Action Port : ActionPort  ActionPortLabel=if(u1 == 1 | u2 == 1)
  Constant2 : Constant  Value=0
  Constant4 : Constant  Value=platformSelection
  Custom Discrete PD (Attitude) : Subsystem
  Custom Discrete PD (X-Position) : Subsystem
  Custom Discrete PD (Y-Position) : Subsystem
  Data Store Write3 : DataStoreWrite  DataStoreName=Float_State
  Desired Px (BLACK) : Constant  Value=home_states_RED(1)  SampleTime=-1
  Desired Px (BLACK)1 : Constant  Value=home_states_RED(2)  SampleTime=-1
  Desired Px (BLACK)2 : Constant  Value=home_states_RED(3)  SampleTime=-1
  Hough Control : Subsystem
  If : If  IfExpression=u1 == 4 | u1 == 5 | u1 == 10 | u1 == 11
  Puck State : Constant
  RED : Subsystem  TreatAsAtomicUnit=on
  RED+ARM : Subsystem  TreatAsAtomicUnit=on
  RED_Fx : DataStoreWrite  DataStoreName=RED_Fx
  RED_Fy : DataStoreWrite  DataStoreName=RED_Fy
  RED_Px : DataStoreRead  DataStoreName=RED_Px
  "RED_Py " : DataStoreRead  DataStoreName=RED_Py
  RED_Rz : DataStoreRead  DataStoreName=RED_Rz
  RED_Tz : DataStoreWrite  DataStoreName=RED_Tz
  RED_Tz_RW1 : DataStoreWrite  DataStoreName=RED_Tz_RW
  Subtract : Sum  Inputs=+-
  Subtract1 : Sum  Inputs=+-
  wires:
  Constant2/1 -> RED_Tz_RW1/1
  Desired Px (BLACK)/1 -> Subtract/1
  Custom Discrete PD (Attitude)/1(Tz) -> RED_Tz/1
  Desired Px (BLACK)2/1 -> Hough Control/1(Ref)
  RED_Rz/1 -> Hough Control/2(Act)
  Desired Px (BLACK)1/1 -> Subtract1/1
  Custom Discrete PD (X-Position)/1(Fx) -> RED_Fx/1
  Subtract/1 -> Custom Discrete PD (X-Position)/1(ex)
  Hough Control/1(Err) -> Custom Discrete PD (Attitude)/1(ez)
  Custom Discrete PD (Y-Position)/1(Fy) -> RED_Fy/1
  RED_Px/1 -> Subtract/2
  "RED_Py "/1 -> Subtract1/2
  Subtract1/1 -> Custom Discrete PD (Y-Position)/1(ey)
  Puck State/1 -> Data Store Write3/1
  If/1 -> RED+ARM/Action
  If/2 -> RED/Action
  Constant4/1 -> If/1

== system Template_v3_08_2020a/Phase #4: Return Home/Is this a simulation? ==
  Constant : Constant  Value=simMode  SampleTime=-1
  isSim : Outport  VectorParamsAs1DForOutWhenUnconnected=off
  wires:
  Constant/1 -> isSim/1

== system Template_v3_08_2020a/Phase #5: Hold Home/Change BLACK Behavior ==
  note: Additional Blocks
  note: PD Control Law - BLACK
  note: A simple PD control law is used here to command the platform to it's initial position, as defined in the initializer.
  note: Additional blocks are stored here.
  Action Port : ActionPort  ActionPortLabel=if(u1 == 2 | u2 == 1)
  BLACK_Fx : DataStoreWrite  DataStoreName=BLACK_Fx
  BLACK_Fy : DataStoreWrite  DataStoreName=BLACK_Fy
  BLACK_Px : DataStoreRead  DataStoreName=BLACK_Px
  "BLACK_Py " : DataStoreRead  DataStoreName=BLACK_Py
  BLACK_Rz : DataStoreRead  DataStoreName=BLACK_Rz
  BLACK_Tz : DataStoreWrite  DataStoreName=BLACK_Tz
  Constant : Constant  Value=home_states_BLACK(1)
  Constant1 : Constant
  Constant2 : Constant  Value=home_states_BLACK(2)
  Constant3 : Constant  Value=home_states_BLACK(3)
  Custom Discrete PD (Attitude) : Subsystem
  Custom Discrete PD (X-Position) : Subsystem
  Custom Discrete PD (Y-Position) : Subsystem
  Data Store Write : DataStoreWrite  DataStoreName=Magnet_State
  Data Store Write3 : DataStoreWrite  DataStoreName=Float_State
  Hough Control : Subsystem
  Puck State : Constant
  Subtract : Sum  Inputs=+-
  Subtract1 : Sum  Inputs=+-
  wires:
  Custom Discrete PD (X-Position)/1(Fx) -> BLACK_Fx/1
  "BLACK_Py "/1 -> Subtract1/2
  Subtract1/1 -> Custom Discrete PD (Y-Position)/1(ey)
  Custom Discrete PD (Y-Position)/1(Fy) -> BLACK_Fy/1
  Constant3/1 -> Hough Control/1(Ref)
  Constant/1 -> Subtract/1
  Constant2/1 -> Subtract1/1
  Subtract/1 -> Custom Discrete PD (X-Position)/1(ex)
  Hough Control/1(Err) -> Custom Discrete PD (Attitude)/1(ez)
  Custom Discrete PD (Attitude)/1(Tz) -> BLACK_Tz/1
  BLACK_Px/1 -> Subtract/2
  BLACK_Rz/1 -> Hough Control/2(Act)
  Puck State/1 -> Data Store Write3/1
  Constant1/1 -> Data Store Write/1

== system Template_v3_08_2020a/Phase #5: Hold Home/Change BLUE Behavior ==
  note: PD Control Law - WHITE
  note: Additional blocks are stored here.
  note: A simple PD control law is used here to command the platform to it's initial position, as defined in the initializer.
  note: Additional Blocks
  Action Port : ActionPort  ActionPortLabel=if(u1 == 3 | u2 == 1)
  BLUE_Fx : DataStoreWrite  DataStoreName=BLUE_Fx
  BLUE_Fy : DataStoreWrite  DataStoreName=BLUE_Fy
  BLUE_Px : DataStoreRead  DataStoreName=BLUE_Px
  "BLUE_Py " : DataStoreRead  DataStoreName=BLUE_Py
  BLUE_Rz : DataStoreRead  DataStoreName=BLUE_Rz
  BLUE_Tz : DataStoreWrite  DataStoreName=BLUE_Tz
  Custom Discrete PD (Attitude) : Subsystem
  Custom Discrete PD (X-Position) : Subsystem
  Custom Discrete PD (Y-Position) : Subsystem
  Data Store Write3 : DataStoreWrite  DataStoreName=Float_State
  Desired Attitude (BLUE) : Constant  Value=home_states_BLUE(3)  SampleTime=-1
  Desired Px (BLUE) : Constant  Value=home_states_BLUE(1)  SampleTime=-1
  Desired Py (BLUE) : Constant  Value=home_states_BLUE(2)  SampleTime=-1
  Hough Control : Subsystem
  Puck State : Constant
  Subtract : Sum  Inputs=+-
  Subtract1 : Sum  Inputs=+-
  wires:
  Puck State/1 -> Data Store Write3/1
  Custom Discrete PD (Y-Position)/1(Fy) -> BLUE_Fy/1
  Custom Discrete PD (X-Position)/1(Fx) -> BLUE_Fx/1
  Subtract1/1 -> Custom Discrete PD (Y-Position)/1(ey)
  "BLUE_Py "/1 -> Subtract1/2
  Desired Px (BLUE)/1 -> Subtract/1
  Hough Control/1(Err) -> Custom Discrete PD (Attitude)/1(ez)
  Subtract/1 -> Custom Discrete PD (X-Position)/1(ex)
  Custom Discrete PD (Attitude)/1(Tz) -> BLUE_Tz/1
  BLUE_Rz/1 -> Hough Control/2(Act)
  Desired Py (BLUE)/1 -> Subtract1/1
  BLUE_Px/1 -> Subtract/2
  Desired Attitude (BLUE)/1 -> Hough Control/1(Ref)

== system Template_v3_08_2020a/Phase #5: Hold Home/Change RED Behavior ==
  note: PD Control Law - RED
  note: Additional Blocks
  note: Additional blocks are stored above. Note that to control attitude using the RW, simply replace RED_Tz with RED_Tz_RW.
  note: A simple PD control law is used here to command the platform to it's home position, as defined in the initializer.
  note: ARM Control Law - RED
  Action Port : ActionPort  ActionPortLabel=if(u1 == 1 | u2 == 1)
  Constant1 : Constant  Value=0
  Constant4 : Constant  Value=platformSelection
  Custom Discrete PD (Attitude) : Subsystem
  Custom Discrete PD (X-Position) : Subsystem
  Custom Discrete PD (Y-Position) : Subsystem
  Data Store Write3 : DataStoreWrite  DataStoreName=Float_State
  Desired Px (BLACK) : Constant  Value=home_states_RED(1)  SampleTime=-1
  Desired Px (BLACK)1 : Constant  Value=home_states_RED(2)  SampleTime=-1
  Desired Px (BLACK)2 : Constant  Value=home_states_RED(3)  SampleTime=-1
  Hough Control : Subsystem
  If : If  IfExpression=u1 == 4 | u1 == 5 | u1 == 10 | u1 == 11
  Puck State : Constant
  RED : Subsystem  TreatAsAtomicUnit=on
  RED+ARM : Subsystem  TreatAsAtomicUnit=on
  RED_Fx : DataStoreWrite  DataStoreName=RED_Fx
  RED_Fy : DataStoreWrite  DataStoreName=RED_Fy
  RED_Px : DataStoreRead  DataStoreName=RED_Px
  "RED_Py " : DataStoreRead  DataStoreName=RED_Py
  RED_Rz : DataStoreRead  DataStoreName=RED_Rz
  RED_Tz : DataStoreWrite  DataStoreName=RED_Tz
  RED_Tz_RW : DataStoreWrite  DataStoreName=RED_Tz_RW
  Subtract : Sum  Inputs=+-
  Subtract1 : Sum  Inputs=+-
  wires:
  Constant1/1 -> RED_Tz_RW/1
  Puck State/1 -> Data Store Write3/1
  Desired Px (BLACK)1/1 -> Subtract1/1
  Custom Discrete PD (Attitude)/1(Tz) -> RED_Tz/1
  "RED_Py "/1 -> Subtract1/2
  RED_Rz/1 -> Hough Control/2(Act)
  Desired Px (BLACK)/1 -> Subtract/1
  Custom Discrete PD (Y-Position)/1(Fy) -> RED_Fy/1
  Subtract1/1 -> Custom Discrete PD (Y-Position)/1(ey)
  Custom Discrete PD (X-Position)/1(Fx) -> RED_Fx/1
  Subtract/1 -> Custom Discrete PD (X-Position)/1(ex)
  Hough Control/1(Err) -> Custom Discrete PD (Attitude)/1(ez)
  Desired Px (BLACK)2/1 -> Hough Control/1(Ref)
  RED_Px/1 -> Subtract/2
  If/1 -> RED+ARM/Action
  If/2 -> RED/Action
  Constant4/1 -> If/1

== system Template_v3_08_2020a/Phase #5: Hold Home/Is this a simulation? ==
  Constant : Constant  Value=simMode  SampleTime=-1
  isSim : Outport  VectorParamsAs1DForOutWhenUnconnected=off
  wires:
  Constant/1 -> isSim/1

== system Template_v3_08_2020a/Phase #6: Stop Floating and Spin Down RW/Change BLACK Behavior ==
  note: At the end of the experiment, the pucks must be turned off.
  note: At the end of the experiment, all thrust and arms movement must cease.
  Action Port : ActionPort  ActionPortLabel=if(u1 == 2 | u2 == 1)
  BLACK_Fx : DataStoreWrite  DataStoreName=BLACK_Fx
  BLACK_Fy : DataStoreWrite  DataStoreName=BLACK_Fy
  BLACK_Tz : DataStoreWrite  DataStoreName=BLACK_Tz
  Constant1 : Constant
  Constant3 : Constant  Value=0
  Constant4 : Constant  Value=0
  Constant5 : Constant  Value=0
  Data Store Write : DataStoreWrite  DataStoreName=Magnet_State
  Data Store Write3 : DataStoreWrite  DataStoreName=Float_State
  Puck State : Constant  Value=0
  wires:
  Constant3/1 -> BLACK_Fx/1
  Constant5/1 -> BLACK_Tz/1
  Constant4/1 -> BLACK_Fy/1
  Puck State/1 -> Data Store Write3/1
  Constant1/1 -> Data Store Write/1

== system Template_v3_08_2020a/Phase #6: Stop Floating and Spin Down RW/Change BLUE Behavior ==
  note: Before getting good data, the platforms must NOT be floating. So, float is set to be "off".
  note: For the initialization phase, we do not want any thrust. Thus, all commanded forces are zero.
  Action Port : ActionPort  ActionPortLabel=if(u1 == 3 | u2 == 1)
  BLUE_Fx : DataStoreWrite  DataStoreName=BLUE_Fx
  BLUE_Fy : DataStoreWrite  DataStoreName=BLUE_Fy
  BLUE_Tz : DataStoreWrite  DataStoreName=BLUE_Tz
  Constant3 : Constant  Value=0
  Constant4 : Constant  Value=0
  Constant5 : Constant  Value=0
  Data Store Write4 : DataStoreWrite  DataStoreName=Float_State
  Puck State : Constant  Value=0
  wires:
  Constant3/1 -> BLUE_Fx/1
  Constant5/1 -> BLUE_Tz/1
  Constant4/1 -> BLUE_Fy/1
  Puck State/1 -> Data Store Write4/1

== system Template_v3_08_2020a/Phase #6: Stop Floating and Spin Down RW/Change RED Behavior ==
  note: At the end of the experiment, the pucks must be turned off.
  note: At the end of the experiment, all thrust and arms movement must cease.
  note: Once the platform has settled, the RW must be slowly desaturated (assuming it has been used).
  Action Port : ActionPort  ActionPortLabel=if(u1 == 1 | u2 == 1)
  Constant{,1..3} (4 alike) : Constant  Value=0
  Data Store Write3 : DataStoreWrite  DataStoreName=Float_State
  Data Store Write4 : DataStoreWrite  DataStoreName=RED_ARM_Control_Mode
  Gain : Gain  Gain=-1
  Puck State : Constant  Value=0
  RED_Fx : DataStoreWrite  DataStoreName=RED_Fx
  RED_Fy : DataStoreWrite  DataStoreName=RED_Fy
  RED_Tz : DataStoreWrite  DataStoreName=RED_Tz
  RED_Tz_RW : DataStoreWrite  DataStoreName=RED_Tz_RW
  RED_dRz_Speed : DataStoreRead  DataStoreName=RED_dRz_RW_Sat
  Saturation : Saturate  UpperLimit=0.005  LowerLimit=-0.005
  wires:
  Constant/1 -> RED_Fx/1
  RED_dRz_Speed/1 -> Gain/1
  Saturation/1 -> RED_Tz_RW/1
  Constant1/1 -> RED_Fy/1
  Gain/1 -> Saturation/1
  Constant2/1 -> RED_Tz/1
  Puck State/1 -> Data Store Write3/1
  Constant3/1 -> Data Store Write4/1

== system Template_v3_08_2020a/Phase #6: Stop Floating and Spin Down RW/Is this a simulation? ==
  Constant : Constant  Value=simMode  SampleTime=-1
  isSim : Outport  VectorParamsAs1DForOutWhenUnconnected=off
  wires:
  Constant/1 -> isSim/1
